simulink model "htg_ad9213"  (R2019a)
settings: Solver=VariableStepAuto  StartTime=0.0  StopTime=500  RelTol=1e-3
libraries: xbsIndex_r4 x33
settings Model: Creator=qwerty40  LastModifiedBy=jackh
settings DataIOCC: ReturnWorkspaceOutputs=off
settings DebuggingCC: ArithmeticOperatorsInVariantConditions=warning
settings SFSimCC: SimUseLocalCustomCode=off
settings RTWCC: RTWUseLocalCustomCode=off
settings CodeAppCC: StateflowObjectComments=on

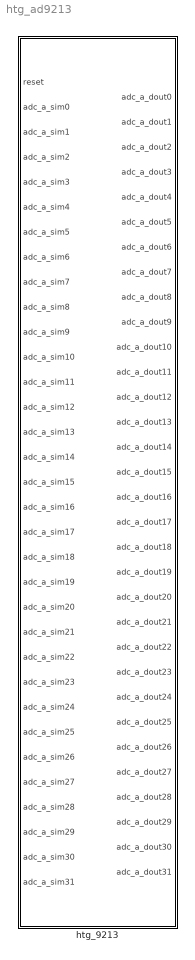
== system htg_ad9213 ==
  htg_9213 : Subsystem  Tag=xps:htg_ad9213  mask(htg_ad9213){use_fmc_a=on, use_fmc_b=off, use_fmc_c=off, use_fmc_d=off, use_uart=off, source_path='', adc_clk_rate=800, sample_period=4}
      mask prompts: use_fmc_a "Use FMC A"; use_fmc_b "Use FMC B"; use_fmc_c "Use FMC C"; use_fmc_d "Use FMC D"; use_uart "Use UART"; source_path "Source code path"; adc_clk_rate "ADC clock rate (MHz)"; sample_period "Sample period"
      mask init:
      | htg_ad9213_mask(gcb, ...
      |     use_fmc_a, ...
      |     use_fmc_b, ...
      |     use_fmc_c, ...
      |     use_fmc_d);

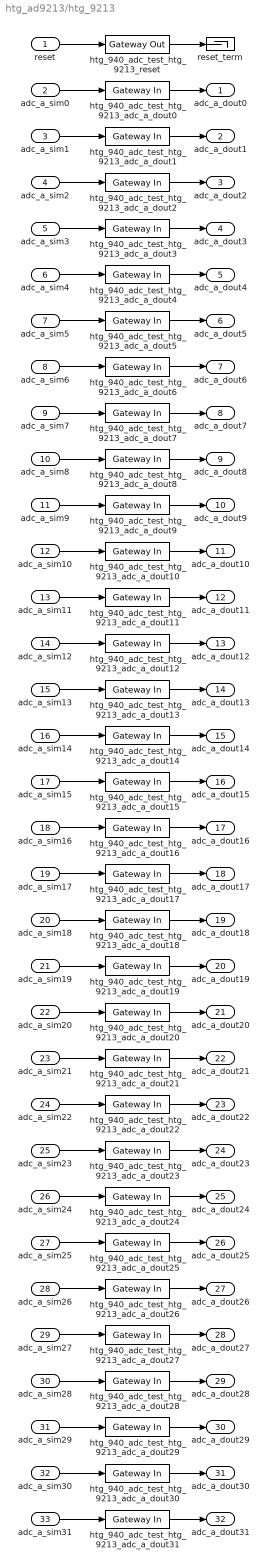
== system htg_ad9213/htg_9213 ==
  reset : Inport
  adc_a_sim0 : Inport  Port=2
  adc_a_sim1 : Inport  Port=3
  adc_a_sim2 : Inport  Port=4
  adc_a_sim3 : Inport  Port=5
  adc_a_sim4 : Inport  Port=6
  adc_a_sim5 : Inport  Port=7
  adc_a_sim6 : Inport  Port=8
  adc_a_sim7 : Inport  Port=9
  adc_a_sim8 : Inport  Port=10
  adc_a_sim9 : Inport  Port=11
  adc_a_sim10 : Inport  Port=12
  adc_a_sim11 : Inport  Port=13
  adc_a_sim12 : Inport  Port=14
  adc_a_sim13 : Inport  Port=15
  adc_a_sim14 : Inport  Port=16
  adc_a_sim15 : Inport  Port=17
  adc_a_sim16 : Inport  Port=18
  adc_a_sim17 : Inport  Port=19
  adc_a_sim18 : Inport  Port=20
  adc_a_sim19 : Inport  Port=21
  adc_a_sim20 : Inport  Port=22
  adc_a_sim21 : Inport  Port=23
  adc_a_sim22 : Inport  Port=24
  adc_a_sim23 : Inport  Port=25
  adc_a_sim24 : Inport  Port=26
  adc_a_sim25 : Inport  Port=27
  adc_a_sim26 : Inport  Port=28
  adc_a_sim27 : Inport  Port=29
  adc_a_sim28 : Inport  Port=30
  adc_a_sim29 : Inport  Port=31
  adc_a_sim30 : Inport  Port=32
  adc_a_sim31 : Inport  Port=33
  htg_940_adc_test_htg_9213_adc_a_dout{0..31} (32 alike) : xbsIndex_r4/Gateway In  gui_display_data_type=Fixed-point  arith_type="Signed  (2's comp)"  n_bits=12  bin_pt=11  preci_type=Single  exp_width=8  frac_width=24  rows=1  columns=1  quantization="Round  (unbiased: +/- Inf)"  overflow=Saturate  period=1  UseAsADC=off  ADCChannel='1'  interface=None  automatic_assignment=on  address_offset=hex2dec('00')  intf_name=''  intf_description=''  default_value=0  timing_constraint=None  locs_specified=off  LOCs={}  io_standard={}  inherit_from_input=off  hdl_port=on  dbl_ovrd=off  block_type=gatewayin
  htg_940_adc_test_htg_9213_reset : xbsIndex_r4/Gateway Out  inherit_from_input=off  hdl_port=on  rows=1  columns=1  UseAsDAC=off  DACChannel='1'  interface=None  automatic_assignment=on  address_offset=hex2dec('00')  intf_name=''  intf_description=''  timing_constraint=None  locs_specified=off  LOCs={}  io_standard={}  block_type=gatewayout
  reset_term : Terminator
  adc_a_dout0 : Outport
  adc_a_dout1 : Outport  Port=2
  adc_a_dout2 : Outport  Port=3
  adc_a_dout3 : Outport  Port=4
  adc_a_dout4 : Outport  Port=5
  adc_a_dout5 : Outport  Port=6
  adc_a_dout6 : Outport  Port=7
  adc_a_dout7 : Outport  Port=8
  adc_a_dout8 : Outport  Port=9
  adc_a_dout9 : Outport  Port=10
  adc_a_dout10 : Outport  Port=11
  adc_a_dout11 : Outport  Port=12
  adc_a_dout12 : Outport  Port=13
  adc_a_dout13 : Outport  Port=14
  adc_a_dout14 : Outport  Port=15
  adc_a_dout15 : Outport  Port=16
  adc_a_dout16 : Outport  Port=17
  adc_a_dout17 : Outport  Port=18
  adc_a_dout18 : Outport  Port=19
  adc_a_dout19 : Outport  Port=20
  adc_a_dout20 : Outport  Port=21
  adc_a_dout21 : Outport  Port=22
  adc_a_dout22 : Outport  Port=23
  adc_a_dout23 : Outport  Port=24
  adc_a_dout24 : Outport  Port=25
  adc_a_dout25 : Outport  Port=26
  adc_a_dout26 : Outport  Port=27
  adc_a_dout27 : Outport  Port=28
  adc_a_dout28 : Outport  Port=29
  adc_a_dout29 : Outport  Port=30
  adc_a_dout30 : Outport  Port=31
  adc_a_dout31 : Outport  Port=32
  wires:
  reset/1 -> htg_940_adc_test_htg_9213_reset/1
  htg_940_adc_test_htg_9213_reset/1 -> reset_term/1
  adc_a_sim0/1 -> htg_940_adc_test_htg_9213_adc_a_dout0/1
  htg_940_adc_test_htg_9213_adc_a_dout0/1 -> adc_a_dout0/1
  adc_a_sim1/1 -> htg_940_adc_test_htg_9213_adc_a_dout1/1
  htg_940_adc_test_htg_9213_adc_a_dout1/1 -> adc_a_dout1/1
  adc_a_sim2/1 -> htg_940_adc_test_htg_9213_adc_a_dout2/1
  htg_940_adc_test_htg_9213_adc_a_dout2/1 -> adc_a_dout2/1
  adc_a_sim3/1 -> htg_940_adc_test_htg_9213_adc_a_dout3/1
  htg_940_adc_test_htg_9213_adc_a_dout3/1 -> adc_a_dout3/1
  adc_a_sim4/1 -> htg_940_adc_test_htg_9213_adc_a_dout4/1
  htg_940_adc_test_htg_9213_adc_a_dout4/1 -> adc_a_dout4/1
  adc_a_sim5/1 -> htg_940_adc_test_htg_9213_adc_a_dout5/1
  htg_940_adc_test_htg_9213_adc_a_dout5/1 -> adc_a_dout5/1
  adc_a_sim6/1 -> htg_940_adc_test_htg_9213_adc_a_dout6/1
  htg_940_adc_test_htg_9213_adc_a_dout6/1 -> adc_a_dout6/1
  adc_a_sim7/1 -> htg_940_adc_test_htg_9213_adc_a_dout7/1
  htg_940_adc_test_htg_9213_adc_a_dout7/1 -> adc_a_dout7/1
  adc_a_sim8/1 -> htg_940_adc_test_htg_9213_adc_a_dout8/1
  htg_940_adc_test_htg_9213_adc_a_dout8/1 -> adc_a_dout8/1
  adc_a_sim9/1 -> htg_940_adc_test_htg_9213_adc_a_dout9/1
  htg_940_adc_test_htg_9213_adc_a_dout9/1 -> adc_a_dout9/1
  adc_a_sim10/1 -> htg_940_adc_test_htg_9213_adc_a_dout10/1
  htg_940_adc_test_htg_9213_adc_a_dout10/1 -> adc_a_dout10/1
  adc_a_sim11/1 -> htg_940_adc_test_htg_9213_adc_a_dout11/1
  htg_940_adc_test_htg_9213_adc_a_dout11/1 -> adc_a_dout11/1
  adc_a_sim12/1 -> htg_940_adc_test_htg_9213_adc_a_dout12/1
  htg_940_adc_test_htg_9213_adc_a_dout12/1 -> adc_a_dout12/1
  adc_a_sim13/1 -> htg_940_adc_test_htg_9213_adc_a_dout13/1
  htg_940_adc_test_htg_9213_adc_a_dout13/1 -> adc_a_dout13/1
  adc_a_sim14/1 -> htg_940_adc_test_htg_9213_adc_a_dout14/1
  htg_940_adc_test_htg_9213_adc_a_dout14/1 -> adc_a_dout14/1
  adc_a_sim15/1 -> htg_940_adc_test_htg_9213_adc_a_dout15/1
  htg_940_adc_test_htg_9213_adc_a_dout15/1 -> adc_a_dout15/1
  adc_a_sim16/1 -> htg_940_adc_test_htg_9213_adc_a_dout16/1
  htg_940_adc_test_htg_9213_adc_a_dout16/1 -> adc_a_dout16/1
  adc_a_sim17/1 -> htg_940_adc_test_htg_9213_adc_a_dout17/1
  htg_940_adc_test_htg_9213_adc_a_dout17/1 -> adc_a_dout17/1
  adc_a_sim18/1 -> htg_940_adc_test_htg_9213_adc_a_dout18/1
  htg_940_adc_test_htg_9213_adc_a_dout18/1 -> adc_a_dout18/1
  adc_a_sim19/1 -> htg_940_adc_test_htg_9213_adc_a_dout19/1
  htg_940_adc_test_htg_9213_adc_a_dout19/1 -> adc_a_dout19/1
  adc_a_sim20/1 -> htg_940_adc_test_htg_9213_adc_a_dout20/1
  htg_940_adc_test_htg_9213_adc_a_dout20/1 -> adc_a_dout20/1
  adc_a_sim21/1 -> htg_940_adc_test_htg_9213_adc_a_dout21/1
  htg_940_adc_test_htg_9213_adc_a_dout21/1 -> adc_a_dout21/1
  adc_a_sim22/1 -> htg_940_adc_test_htg_9213_adc_a_dout22/1
  htg_940_adc_test_htg_9213_adc_a_dout22/1 -> adc_a_dout22/1
  adc_a_sim23/1 -> htg_940_adc_test_htg_9213_adc_a_dout23/1
  htg_940_adc_test_htg_9213_adc_a_dout23/1 -> adc_a_dout23/1
  adc_a_sim24/1 -> htg_940_adc_test_htg_9213_adc_a_dout24/1
  htg_940_adc_test_htg_9213_adc_a_dout24/1 -> adc_a_dout24/1
  adc_a_sim25/1 -> htg_940_adc_test_htg_9213_adc_a_dout25/1
  htg_940_adc_test_htg_9213_adc_a_dout25/1 -> adc_a_dout25/1
  adc_a_sim26/1 -> htg_940_adc_test_htg_9213_adc_a_dout26/1
  htg_940_adc_test_htg_9213_adc_a_dout26/1 -> adc_a_dout26/1
  adc_a_sim27/1 -> htg_940_adc_test_htg_9213_adc_a_dout27/1
  htg_940_adc_test_htg_9213_adc_a_dout27/1 -> adc_a_dout27/1
  adc_a_sim28/1 -> htg_940_adc_test_htg_9213_adc_a_dout28/1
  htg_940_adc_test_htg_9213_adc_a_dout28/1 -> adc_a_dout28/1
  adc_a_sim29/1 -> htg_940_adc_test_htg_9213_adc_a_dout29/1
  htg_940_adc_test_htg_9213_adc_a_dout29/1 -> adc_a_dout29/1
  adc_a_sim30/1 -> htg_940_adc_test_htg_9213_adc_a_dout30/1
  htg_940_adc_test_htg_9213_adc_a_dout30/1 -> adc_a_dout30/1
  adc_a_sim31/1 -> htg_940_adc_test_htg_9213_adc_a_dout31/1
  htg_940_adc_test_htg_9213_adc_a_dout31/1 -> adc_a_dout31/1
